simulink model "prob6"  (R2020b)
settings: Solver=VariableStepAuto  StartTime=0.0  StopTime=10  MaxStep=0.001  RelTol=1e-3
model workspace: external: MATLAB File C:\Users\deves\MATLAB\Projects\problem6\data6.m (data not in the file)
settings Model: Creator=deves  LastModifiedBy=deves

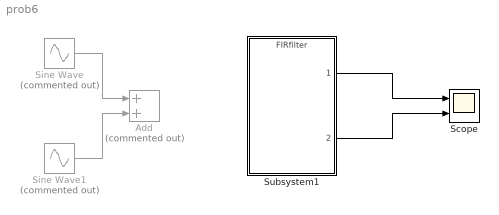
== system prob6 ==
  Add : Sum  Commented=on
  Scope : Scope  NumInputPorts=2
  Sine Wave : Sin  Commented=on  SampleTime=0
  Sine Wave1 : Sin  Commented=on  Frequency=100  SampleTime=0
  Subsystem1 : ModelReference  ModelNameDialog=FIRfilter  SimulationMode=Normal  ModelReferenceVersion=1.6
  wires:
  Subsystem1/1 -> Scope/1
  Subsystem1/2 -> Scope/2
  Sine Wave/1 -> Add/1
  Sine Wave1/1 -> Add/2
